simulink model "SimPract2"  (R2018a)
settings: Solver=ode45  StartTime=0.0  StopTime=0.1  RelTol=1e-9
values from neighbouring files (symbols this model uses):
  J = 800*D^4*L*0.1    (= 2.3808e-07)    [Pract2.m]
  Kf = (U-Ra*In)/wn    (= 0.0412529612494)    [Pract2.m]
  La = 0.5*U/In/wn    (= 0.102313891988)    [Pract2.m]
  M0 = M - Mn    (= 0.00665082914984)    [Pract2.m]
  Mn = 4.9e-3    (= 0.0049)    [Pract2.m]
  Ra = U/Ip    (= 27)    [Pract2.m]
  U = 27    [Pract2.m]
settings Model: Creator=dirlak  LastModifiedBy=dirlak

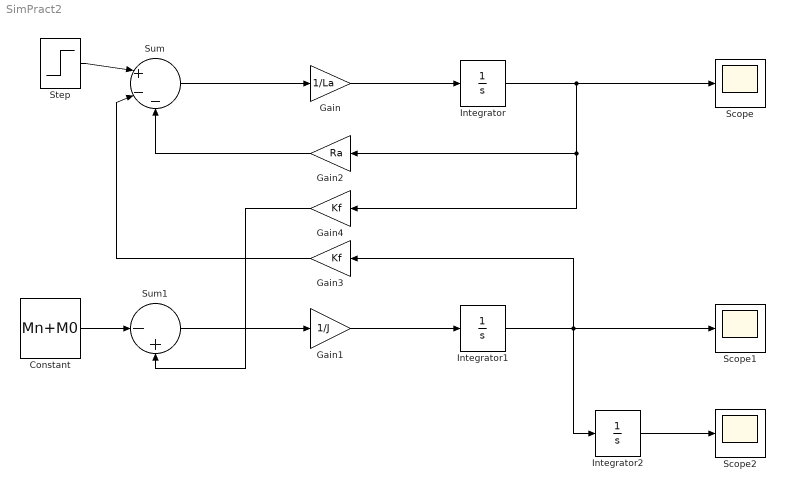
== system SimPract2 ==
  Constant : Constant  Value=Mn+M0
  Gain : Gain  Gain=1/La
  Gain1 : Gain  Gain=1/J
  Gain2 : Gain  Gain=Ra
  Gain3 : Gain  Gain=Kf
  Gain4 : Gain  Gain=Kf
  Integrator : Integrator
  Integrator1 : Integrator
  Integrator2 : Integrator
  Scope : Scope
  Scope1 : Scope
  Scope2 : Scope
  Step : Step  Time=0  After=U  SampleTime=0
  Sum : Sum  Inputs=|+--
  Sum1 : Sum  Inputs=|-+
  wires:
  Sum/1 -> Gain/1
  Gain/1 -> Integrator/1
  Step/1 -> Sum/1
  Constant/1 -> Sum1/1
  Sum1/1 -> Gain1/1
  Gain1/1 -> Integrator1/1
  Integrator1/1 -> Integrator2/1, Scope1/1, Gain3/1
  Gain2/1 -> Sum/3
  Gain3/1 -> Sum/2
  Integrator/1 -> Gain4/1, Gain2/1, Scope/1
  Gain4/1 -> Sum1/2
  Integrator2/1 -> Scope2/1
